simulink model "Ackermann_UGV_Exp"  (R2024a)
settings: Solver=FixedStepAuto  StartTime=0.0  StopTime=300  FixedStep=0.1  MaxStep=0.1  RelTol=1e-3
undefined symbols (not defined in the file or in its folder): Angular, Linear
libraries: robotlib x6, robotcorelib x3
settings Model: Creator=qiaoyike  LastModifiedBy=qiaoyike
settings OptimizationCC: EnhancedBackFolding=on  PassReuseOutputArgsAs=Individual arguments  ZeroExternalMemoryAtStartup=off  ZeroInternalMemoryAtStartup=off  MaxStackSize=64  OptimizeBlockOrder=speed  DifferentSizesBufferReuse=on  OptimizationCustomize=off  EfficientTunableParamExpr=on
settings DebuggingCC: ParameterTunabilityLossMsg=error
settings HardwareCC: ProdBitPerPointer=32  ProdBitPerSizeT=32  ProdBitPerPtrDiffT=32  ProdLargestAtomicFloat=None  ProdIntDivRoundTo=Undefined  ProdEndianess=Unspecified  ProdWordSize=32  ProdHWDeviceType=Generic->Unspecified (assume 32-bit Generic)
settings SFSimCC: MATLABDynamicMemAlloc=off
settings RTWCC: Description=Embedded Coder  SystemTargetFile=ert.tlc  HardwareBoard=Robot Operating System (ROS)  TLCOptions="-aInlineSetEventsForThisBaseRateFcn=TLC_FALSE -aSuppressMultiTaskScheduler=TLC_FALSE  -aRateBasedStepFcn=0"  TemplateMakefile=ert_default_tmf  Toolchain=Catkin  TargetLang=C++  GPUComputeCapability=3.5
settings CodeAppCC: ForceParamTrailComments=on  IgnoreCustomStorageClasses=off  OperatorAnnotations=on  SimulinkDataObjDesc=on  SFDataObjDesc=on  InsertBlockDesc=on
settings ERTTargetCC: SupportNonInlinedSFcns=on  ERTCustomFileTemplate=rostime_codertarget_file_process.tlc

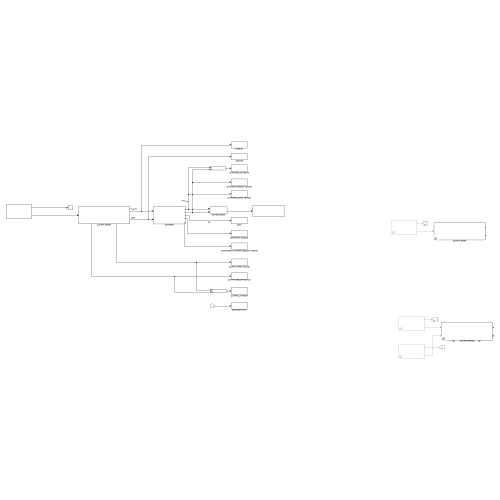
[thumbnail: Simulink's stored preview of the top-level diagram]
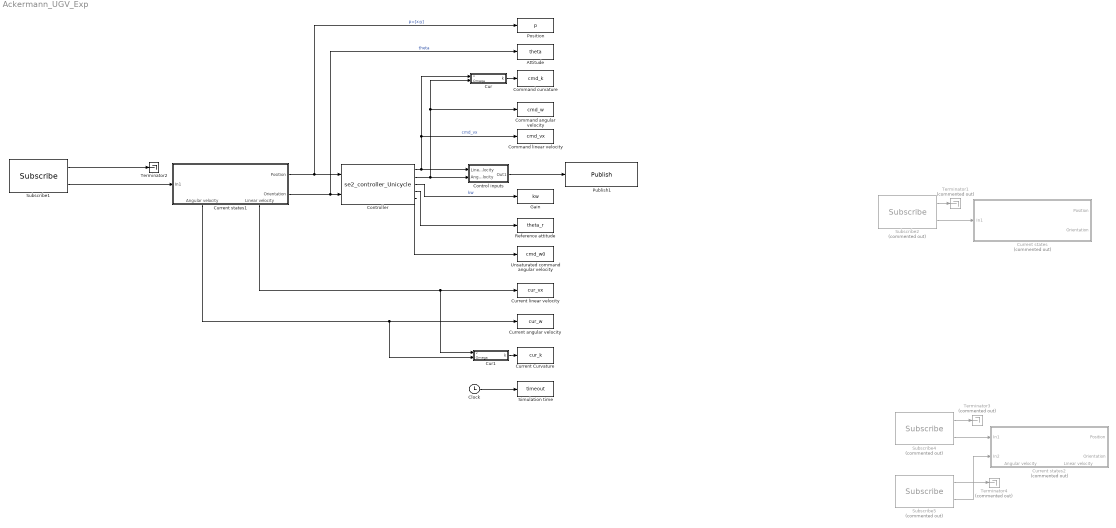
== system Ackermann_UGV_Exp ==
  Attitude : ToWorkspace  VariableName=theta  SampleTime=-1
  Clock : Clock
  Command angular velocity : ToWorkspace  VariableName=cmd_w  SampleTime=-1
  Command curvature : ToWorkspace  VariableName=cmd_k  SampleTime=-1
  Command linear velocity : ToWorkspace  VariableName=cmd_vx  SampleTime=-1
  Control inputs : Subsystem
  Controller : M-S-Function  FunctionName=se2_controller_Unicycle  Parameters=pd,theta_d,rho,v_max,k1,k2,k3  mask{pd=[29.1199745512436;2.80693663090782], theta_d=2.618, rho=0.6, v_max=1, k1=4, k2=8, k3=12}
      mask prompts: pd "Desired posistion [xd;yd]"; theta_d "Desired orientaion in S"; rho "Minimal turning radius"; v_max "Maximum speed"; k1 "CVF parameters k1"; k2 "CVF parameters k2"; k3 "CVF parameters k3"
      mask DialogControl ParameterGroupVar Prompt: 参数
  Cur : MATLAB Function  TreatAsAtomicUnit=on
  Cur1 : MATLAB Function  TreatAsAtomicUnit=on
  Current Curvature : ToWorkspace  VariableName=cur_k  SampleTime=-1
  Current angular velocity : ToWorkspace  VariableName=cur_w  SampleTime=-1
  Current linear velocity : ToWorkspace  VariableName=cur_vx  SampleTime=-1
  Current states : Subsystem  Commented=on
  Current states1 : Subsystem
      settings: PortSchema="{\"entries\":[{\"content\":{\"sides\":[{\"content\":{\"connectorIds\":[\"In1\"]},\"type\":\"ConnectorPlacement.EquallySpacedRectSide\",\"uuid\":\"3a937533-5ac1-47a3-a799-e449f50df633\"},{\"content\":{\"connectorIds\":[\"Out1\",\"Out2\"],\"side\":\"RIGHT\"},\"type\":\"ConnectorPlacement.EquallySpacedRectSide\",\"uuid\":\"28bb4fea-7ea7-48a5-8e7f-13c0477b58b8\"},{\"content\":{\"side\":\"TOP\"},\"type\":\"ConnectorPlacement.EquallySpacedRectSide\",\"uuid\":\"2c556cfe-7bae-48c5-ad5c-7e027ad6d452\"},{\"content\":{\"connectorIds\":[\"Out3\",\"Out4\"],\"side\":\"BOTTOM\"},\"type\":\"ConnectorPlacement.EquallySpacedRectSide\",\"uuid\":\"3229fbf1-2b1c-41ec-8c16-a53d6dc3e59b\"}]},\"type\":\"ConnectorPlacement.EquallySpacedConnector\",\"uuid\":\"d4878a67-c8e4-4d59-ba30-c1e033a78009\"}],\"packageUris\":[\"http://schema.mathworks.com/mf0/Connector/R2020b\"],\"version\":\"1.0\"}"
  Current states2 : Subsystem  Commented=on
      settings: PortSchema="{\"entries\":[{\"content\":{\"sides\":[{\"content\":{\"connectorIds\":[\"In1\",\"In2\"]},\"type\":\"ConnectorPlacement.EquallySpacedRectSide\",\"uuid\":\"5d7394a5-d76f-447d-90fe-ec60b78a0a1b\"},{\"content\":{\"connectorIds\":[\"Out1\",\"Out2\"],\"side\":\"RIGHT\"},\"type\":\"ConnectorPlacement.EquallySpacedRectSide\",\"uuid\":\"5edace55-6d81-420f-a564-ef97bbacc503\"},{\"content\":{\"side\":\"TOP\"},\"type\":\"ConnectorPlacement.EquallySpacedRectSide\",\"uuid\":\"1762584b-5caf-4f6a-a1bf-d951c1c80abd\"},{\"content\":{\"connectorIds\":[\"Out3\",\"Out4\"],\"side\":\"BOTTOM\"},\"type\":\"ConnectorPlacement.EquallySpacedRectSide\",\"uuid\":\"9c178813-a4de-4f00-b500-14a0fce509f6\"}]},\"type\":\"ConnectorPlacement.EquallySpacedConnector\",\"uuid\":\"630df891-3755-42e6-b32a-f72b4379b4d6\"}],\"packageUris\":[\"http://schema.mathworks.com/mf0/Connector/R2020b\"],\"version\":\"1.0\"}"
  Gain : ToWorkspace  VariableName=kw  SampleTime=-1
  Position : ToWorkspace  VariableName=p  SampleTime=-1
  Publish1 : robotlib/Publish  topicSource=Select from ROS network  topic=/cmd_vel  messageType=geometry_msgs/Twist  legacyBusStruct=off  messageQueueLength=100
  Reference attitude : ToWorkspace  VariableName=theta_r  SampleTime=-1
  Simulation time : ToWorkspace  VariableName=timeout  SampleTime=-1
  Subscribe1 : robotlib/Subscribe  topicSource=Select from ROS network  topic=/odom_mocap  messageType=nav_msgs/Odometry  SampleTime=0.1  legacyBusStruct=off  messageQueueLength=1
  Subscribe2 : robotlib/Subscribe  Commented=on  topicSource=Select from ROS network  topic=/vrpn_client_node/ugv3/pose  messageType=geometry_msgs/PoseStamped  SampleTime=0.1  legacyBusStruct=off  messageQueueLength=1
  Subscribe4 : robotlib/Subscribe  Commented=on  topicSource=Select from ROS network  topic=/vrpn_client_node/limo/pose  messageType=geometry_msgs/PoseStamped  SampleTime=0.1  legacyBusStruct=off  messageQueueLength=1
  Subscribe5 : robotlib/Subscribe  Commented=on  topicSource=Select from ROS network  topic=/vrpn_client_node/limo/twist  messageType=geometry_msgs/TwistStamped  SampleTime=0.1  legacyBusStruct=off  messageQueueLength=1
  Terminator1 : Terminator  Commented=on
  Terminator2 : Terminator
  Terminator3 : Terminator  Commented=on
  Terminator4 : Terminator  Commented=on
  Unsaturated command angular velocity : ToWorkspace  VariableName=cmd_w0  SampleTime=-1
  wires:
  Cur/1(k) -> Command curvature/1
  Control inputs/1(Out1) -> Publish1/1
  Subscribe2/2 -> Current states/1(In1)
  Controller/1 -> Control inputs/1(Linear velocity), Cur/1(v), Command linear velocity/1  "cmd_vx"
  Controller/2 -> Control inputs/2(Angular velocity), Cur/2(Omega), Command angular velocity/1
  Controller/3 -> Gain/1  "kw"
  Clock/1 -> Simulation time/1
  Cur1/1(k) -> Current Curvature/1
  Controller/4 -> Reference attitude/1
  Subscribe2/1 -> Terminator1/1
  Controller/5 -> Unsaturated command angular velocity/1
  Current states1/1(Position) -> Position/1, Controller/1  "p=[x;y]"
  Current states1/2(Orientation) -> Attitude/1, Controller/2  "theta"
  Current states1/4(Linear velocity) -> Cur1/1(v), Current linear velocity/1
  Current states1/3(Angular velocity) -> Cur1/2(Omega), Current angular velocity/1
  Subscribe1/1 -> Terminator2/1
  Subscribe1/2 -> Current states1/1(In1)
  Subscribe5/2 -> Current states2/2(In2)
  Subscribe5/1 -> Terminator4/1
  Subscribe4/1 -> Terminator3/1
  Subscribe4/2 -> Current states2/1(In1)

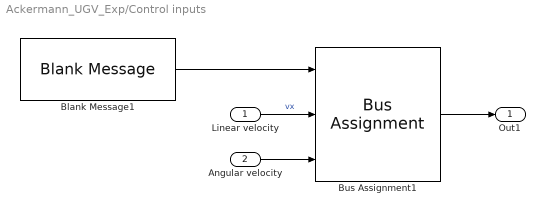
== system Ackermann_UGV_Exp/Control inputs ==
  Linear velocity : Inport
  Angular velocity : Inport  Port=2
  Blank Message1 : robotlib/Blank Message  messageClass=Message  entityType=geometry_msgs/Twist  messageType=geometry_msgs/Twist  SampleTime=inf  legacyBusStruct=off
  Bus Assignment1 : BusAssignment  AssignedSignals=Linear.X,Angular.Z
  Out1 : Outport
  wires:
  Blank Message1/1 -> Bus Assignment1/1
  Bus Assignment1/1 -> Out1/1
  Angular velocity/1 -> Bus Assignment1/3
  Linear velocity/1 -> Bus Assignment1/2  "vx"

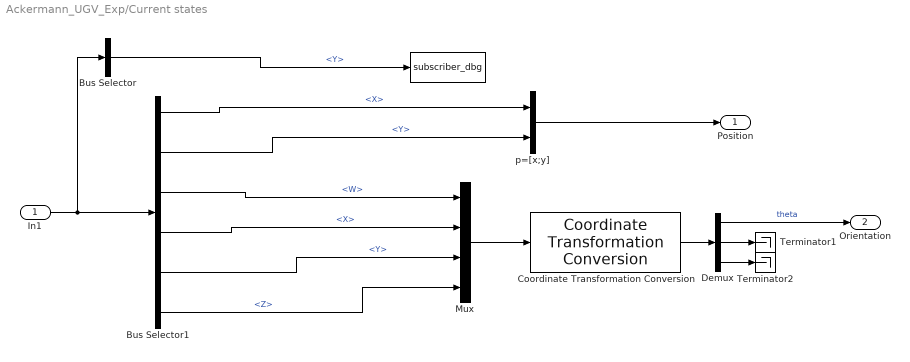
== system Ackermann_UGV_Exp/Current states ==
  In1 : Inport
  " " : ToWorkspace  VariableName=subscriber_dbg  SampleTime=-1
  Bus Selector : BusSelector  OutputSignals=Pose.Position.Y
  Bus Selector1 : BusSelector  OutputSignals=Pose.Position.X,Pose.Position.Y,Pose.Orientation.W,Pose.Orientation.X,Pose.Orientation.Y,Pose.Orientation.Z
  Coordinate Transformation Conversion : robotcorelib/Coordinate Transformation Conversion  InputRepresentation=Quaternion  InputEulerSequence=ZYX  ShowTrVecInputPort=on  OutputRepresentation=Euler Angles  OutputEulerSequence=ZYX  ShowTrVecOutputPort=on  SimulateUsing=Interpreted execution
  Demux : Demux  Outputs=3
  Mux : Mux
  Terminator1 : Terminator
  Terminator2 : Terminator
  p=[x;y] : Mux  Inputs=2
  Position : Outport
  Orientation : Outport  Port=2  PortDimensions=1
  wires:
  Bus Selector1/3 -> Mux/1  "<W>"
  Bus Selector1/5 -> Mux/3  "<Y>"
  Bus Selector1/4 -> Mux/2  "<X>"
  Bus Selector1/6 -> Mux/4  "<Z>"
  Coordinate Transformation Conversion/1 -> Demux/1
  Demux/3 -> Terminator2/1
  Bus Selector1/2 -> p=[x;y]/2  "<Y>"
  Bus Selector1/1 -> p=[x;y]/1  "<X>"
  Demux/2 -> Terminator1/1
  Mux/1 -> Coordinate Transformation Conversion/1
  p=[x;y]/1 -> Position/1
  Demux/1 -> Orientation/1  "theta"
  In1/1 -> Bus Selector/1, Bus Selector1/1
  Bus Selector/1 -> " "/1  "<Y>"

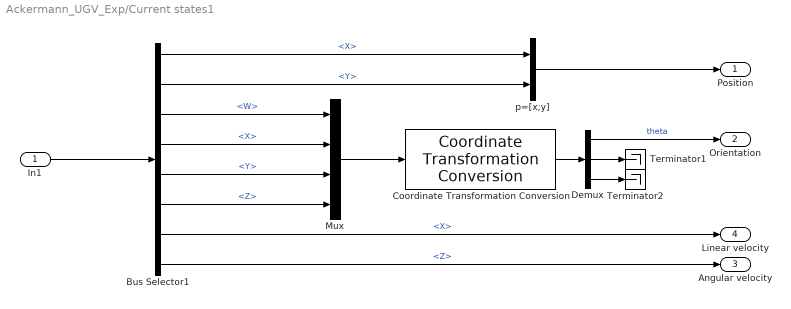
== system Ackermann_UGV_Exp/Current states1 ==
  In1 : Inport
  Bus Selector1 : BusSelector  OutputSignals=Pose.Pose.Position.X,Pose.Pose.Position.Y,Pose.Pose.Orientation.W,Pose.Pose.Orientation.X,Pose.Pose.Orientation.Y,Pose.Pose.Orientation.Z,Twist.Twist.Linear.X,Twist.Twist.Angular.Z
  Coordinate Transformation Conversion : robotcorelib/Coordinate Transformation Conversion  InputRepresentation=Quaternion  InputEulerSequence=ZYX  ShowTrVecInputPort=on  OutputRepresentation=Euler Angles  OutputEulerSequence=ZYX  ShowTrVecOutputPort=on  SimulateUsing=Interpreted execution
  Demux : Demux  Outputs=3
  Mux : Mux
  Terminator1 : Terminator
  Terminator2 : Terminator
  p=[x;y] : Mux  Inputs=2
  Position : Outport
  Orientation : Outport  Port=2  PortDimensions=1
  Angular velocity : Outport  Port=3
  Linear velocity : Outport  Port=4
  wires:
  Bus Selector1/3 -> Mux/1  "<W>"
  Bus Selector1/5 -> Mux/3  "<Y>"
  Bus Selector1/4 -> Mux/2  "<X>"
  Bus Selector1/6 -> Mux/4  "<Z>"
  Coordinate Transformation Conversion/1 -> Demux/1
  Demux/3 -> Terminator2/1
  Bus Selector1/2 -> p=[x;y]/2  "<Y>"
  Bus Selector1/1 -> p=[x;y]/1  "<X>"
  Demux/2 -> Terminator1/1
  Mux/1 -> Coordinate Transformation Conversion/1
  In1/1 -> Bus Selector1/1
  p=[x;y]/1 -> Position/1
  Demux/1 -> Orientation/1  "theta"
  Bus Selector1/7 -> Linear velocity/1  "<X>"
  Bus Selector1/8 -> Angular velocity/1  "<Z>"

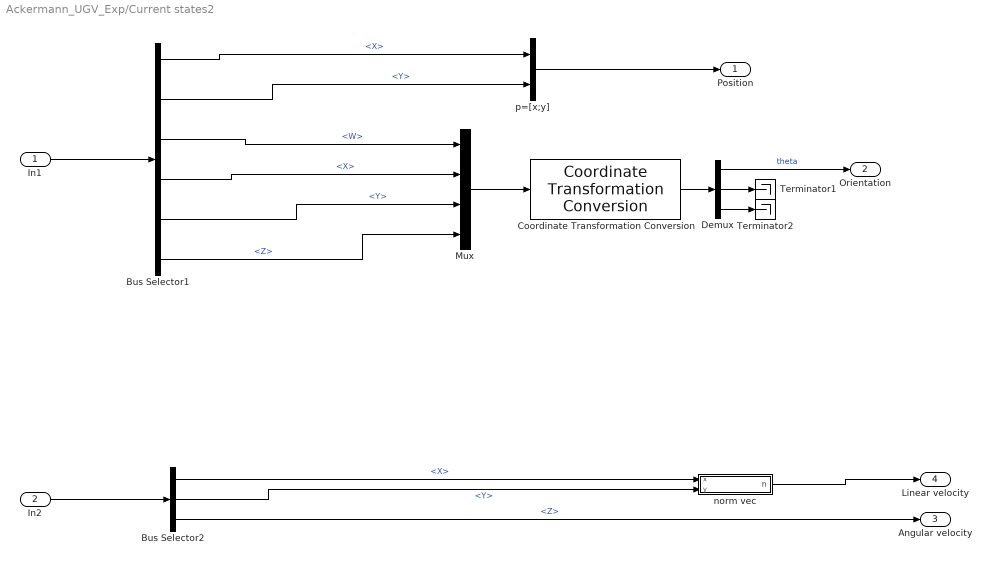
== system Ackermann_UGV_Exp/Current states2 ==
  In1 : Inport
  In2 : Inport  Port=2
  Bus Selector1 : BusSelector  OutputSignals=Pose.Position.X,Pose.Position.Y,Pose.Orientation.W,Pose.Orientation.X,Pose.Orientation.Y,Pose.Orientation.Z
  Bus Selector2 : BusSelector  OutputSignals=Twist.Linear.X,Twist.Linear.Y,Twist.Angular.Z
  Coordinate Transformation Conversion : robotcorelib/Coordinate Transformation Conversion  InputRepresentation=Quaternion  InputEulerSequence=ZYX  ShowTrVecInputPort=on  OutputRepresentation=Euler Angles  OutputEulerSequence=ZYX  ShowTrVecOutputPort=on  SimulateUsing=Interpreted execution
  Demux : Demux  Outputs=3
  Mux : Mux
  Terminator1 : Terminator
  Terminator2 : Terminator
  norm vec : MATLAB Function  TreatAsAtomicUnit=on
  p=[x;y] : Mux  Inputs=2
  Position : Outport
  Orientation : Outport  Port=2  PortDimensions=1
  Angular velocity : Outport  Port=3
  Linear velocity : Outport  Port=4
  wires:
  Bus Selector1/3 -> Mux/1  "<W>"
  Bus Selector1/5 -> Mux/3  "<Y>"
  Bus Selector1/4 -> Mux/2  "<X>"
  Bus Selector1/6 -> Mux/4  "<Z>"
  Coordinate Transformation Conversion/1 -> Demux/1
  Demux/3 -> Terminator2/1
  Bus Selector1/2 -> p=[x;y]/2  "<Y>"
  Bus Selector1/1 -> p=[x;y]/1  "<X>"
  Demux/2 -> Terminator1/1
  Mux/1 -> Coordinate Transformation Conversion/1
  p=[x;y]/1 -> Position/1
  Demux/1 -> Orientation/1  "theta"
  In1/1 -> Bus Selector1/1
  In2/1 -> Bus Selector2/1
  Bus Selector2/3 -> Angular velocity/1  "<Z>"
  Bus Selector2/1 -> norm vec/1(x)  "<X>"
  Bus Selector2/2 -> norm vec/2(y)  "<Y>"
  norm vec/1(n) -> Linear velocity/1

== matlab function Ackermann_UGV_Exp/Cur ==
  data: v input; k output; Omega input
function k = k(v,Omega)
k = norm(Omega)/norm(v);

== matlab function Ackermann_UGV_Exp/Current states2/norm vec ==
  data: x input; n output; y input
function n = norm_vec(x,y)
n = sqrt(x^2+y^2);

== matlab function Ackermann_UGV_Exp/Cur1 ==
  data: v input; k output; Omega input
function k = k(v,Omega)
k = norm(Omega)/norm(v);
